simulink model "RI_PMDC_PI_Z"  (R2013b)
settings: Solver=ode45  StartTime=0.0  StopTime=1  MaxStep=tau_RL/10/25  RelTol=1e-3
InitFcn:
  | % Villamos áramköri rész
  | R = 1.76;
  | L = 658e-6;
  | 
  | % Mágneskör
  | k_T = 68.3e-3;
  | k_E = 68.3e-3;
  | 
  | % Forgó részrendszer
  | J = 99.5e-7;
  | B = 5.7301e-6;
  | 
  | % A belső áramszabályzókör hangolása
  | K_RL = 1/R;
  | tau_RL = L/R;
  | 
  | % ZPK
  | T_I_RL_ZPK = tau_RL;
  | K_PI_RL_ZPK = 1/K_RL * 10;
  | 
  | % MRZK
  | xi_CL_RL = 1;
  | tau_CL_RL = tau_RL/10;
  | 
  | K_PI_RL_MRZK = (2*xi_CL_RL*tau_RL - tau_CL_RL)/(K_RL*tau_CL_RL);
  | T_I_RL_MRZK = (2*xi_CL_RL*tau_RL - tau_CL_RL)*tau_CL_RL/tau_RL;
  | 
  | % A külső szögsebesség-szabályzókör hangolása
  | K_JB = k_T/B;
  | tau_JB = J/B;
  | 
  | % ZPK
  | T_I_JB_ZPK = tau_JB;
  | K_PI_JB_ZPK = 1/K_JB * 2000;
  | 
  | % MRZK
  | xi_CL_JB = 2;
  | tau_CL_JB = tau_JB/2000;
  | 
  | K_PI_JB_MRZK = (2*xi_CL_JB*tau_JB - tau_CL_JB)/(K_JB*tau_CL_JB);
  | T_I_JB_MRZK = (2*xi_CL_JB*tau_JB - tau_CL_JB)*tau_CL_JB/tau_JB;
libraries: RI_MK x6
settings Model: Creator=Szalay  LastModifiedBy=Szalay

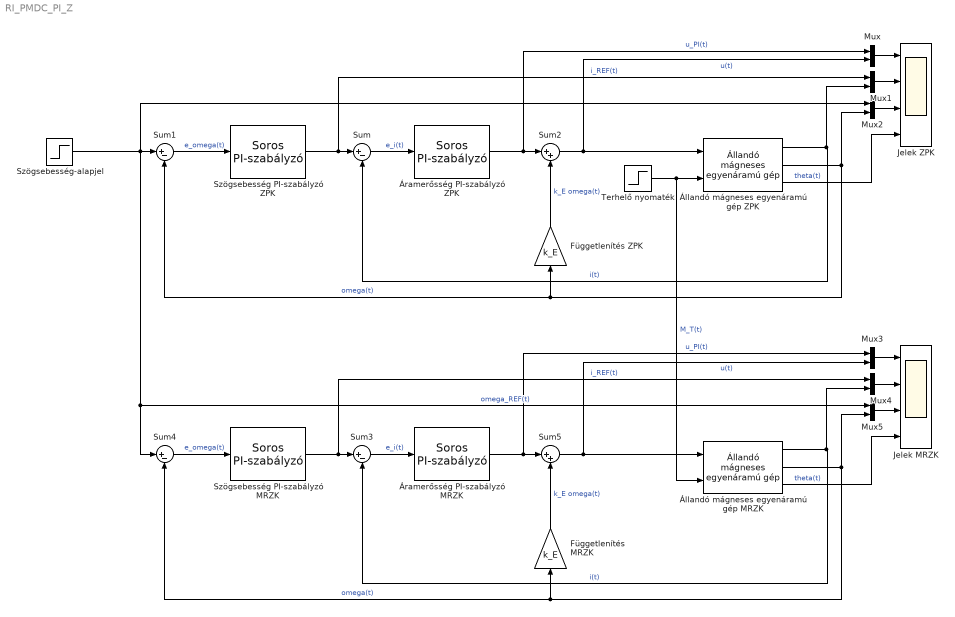
== system RI_PMDC_PI_Z ==
  Függetlenítés MRZK : Gain  Gain=k_E
  Függetlenítés ZPK : Gain  Gain=k_E
  Jelek MRZK : Scope  NumInputPorts=4
      settings: ShowLegends=on  TimeRange=0.5  YMin=-150~-6~-400~0  YMax=150~8~300~40
  Jelek ZPK : Scope  NumInputPorts=4
      settings: ShowLegends=on  TimeRange=0.5  YMin=-150~-6~-400~0  YMax=150~8~300~40
  Mux{,1..5} (6 alike) : Mux  Inputs=2
  Sum{,1,3..4} (4 alike) : Sum  Inputs=|+-
  Sum2 : Sum  Inputs=|++
  Sum5 : Sum  Inputs=|++
  Szögsebesség PI-szabályzó MRZK : RI_MK/Soros PI-szabályzó  K_PI=K_PI_JB_MRZK  T_I=T_I_JB_MRZK
  Szögsebesség PI-szabályzó ZPK : RI_MK/Soros PI-szabályzó  K_PI=K_PI_JB_ZPK  T_I=T_I_JB_ZPK
  Szögsebesség-alapjel : Step  Time=50e-3  After=300  SampleTime=0
  Terhelő nyomaték : Step  Time=250e-3  After=100e-3  SampleTime=0
  Állandó mágneses egyenáramú gép MRZK : RI_MK/Állandó mágneses egyenáramú gép  R=R  L=L  k_T=k_T  k_E=k_E  J=J  B=B  i_0=0  omega_0=0  theta_0=0
  Állandó mágneses egyenáramú gép ZPK : RI_MK/Állandó mágneses egyenáramú gép  R=R  L=L  k_T=k_T  k_E=k_E  J=J  B=B  i_0=0  omega_0=0  theta_0=0
  Áramerősség PI-szabályzó MRZK : RI_MK/Soros PI-szabályzó  K_PI=K_PI_RL_MRZK  T_I=T_I_RL_MRZK
  Áramerősség PI-szabályzó ZPK : RI_MK/Soros PI-szabályzó  K_PI=K_PI_RL_ZPK  T_I=T_I_RL_ZPK
  wires:
  Sum1/1 -> Szögsebesség PI-szabályzó ZPK/1  "e_omega(t)"
  Szögsebesség PI-szabályzó ZPK/1 -> Mux1/1, Sum/1  "i_REF(t)"
  Sum/1 -> Áramerősség PI-szabályzó ZPK/1  "e_i(t)"
  Áramerősség PI-szabályzó ZPK/1 -> Mux/1, Sum2/1  "u_PI(t)"
  Sum2/1 -> Állandó mágneses egyenáramú gép ZPK/1, Mux/2  "u(t)"
  Állandó mágneses egyenáramú gép ZPK/1 -> Mux1/2, Sum/2  "i(t)"
  Állandó mágneses egyenáramú gép ZPK/2 -> Mux2/2, Sum1/2, Függetlenítés ZPK/1  "omega(t)"
  Függetlenítés ZPK/1 -> Sum2/2  "k_E omega(t)"
  Mux/1 -> Jelek ZPK/1
  Mux1/1 -> Jelek ZPK/2
  Mux2/1 -> Jelek ZPK/3
  Állandó mágneses egyenáramú gép ZPK/3 -> Jelek ZPK/4  "theta(t)"
  Sum4/1 -> Szögsebesség PI-szabályzó MRZK/1  "e_omega(t)"
  Szögsebesség PI-szabályzó MRZK/1 -> Mux4/1, Sum3/1  "i_REF(t)"
  Sum3/1 -> Áramerősség PI-szabályzó MRZK/1  "e_i(t)"
  Áramerősség PI-szabályzó MRZK/1 -> Mux3/1, Sum5/1  "u_PI(t)"
  Sum5/1 -> Állandó mágneses egyenáramú gép MRZK/1, Mux3/2  "u(t)"
  Állandó mágneses egyenáramú gép MRZK/1 -> Mux4/2, Sum3/2  "i(t)"
  Állandó mágneses egyenáramú gép MRZK/2 -> Mux5/2, Sum4/2, Függetlenítés MRZK/1  "omega(t)"
  Függetlenítés MRZK/1 -> Sum5/2  "k_E omega(t)"
  Szögsebesség-alapjel/1 -> Sum4/1, Mux5/1, Mux2/1, Sum1/1  "omega_REF(t)"
  Mux3/1 -> Jelek MRZK/1
  Mux4/1 -> Jelek MRZK/2
  Mux5/1 -> Jelek MRZK/3
  Állandó mágneses egyenáramú gép MRZK/3 -> Jelek MRZK/4  "theta(t)"
  Terhelő nyomaték/1 -> Állandó mágneses egyenáramú gép MRZK/2, Állandó mágneses egyenáramú gép ZPK/2  "M_T(t)"
